simulink model "Signal_Generator"  (R2018a)
settings: Solver=VariableStepAuto  StartTime=0.0  StopTime=0.5  RelTol=1e-3
libraries: simulink x20, commrflib2 x4, commsynccomp2 x3
settings Model: Creator=Alam  LastModifiedBy=Administrator
settings CodeAppCC: StateflowObjectComments=on
settings SimscapeCC: SimscapeNormalizeSystem=off

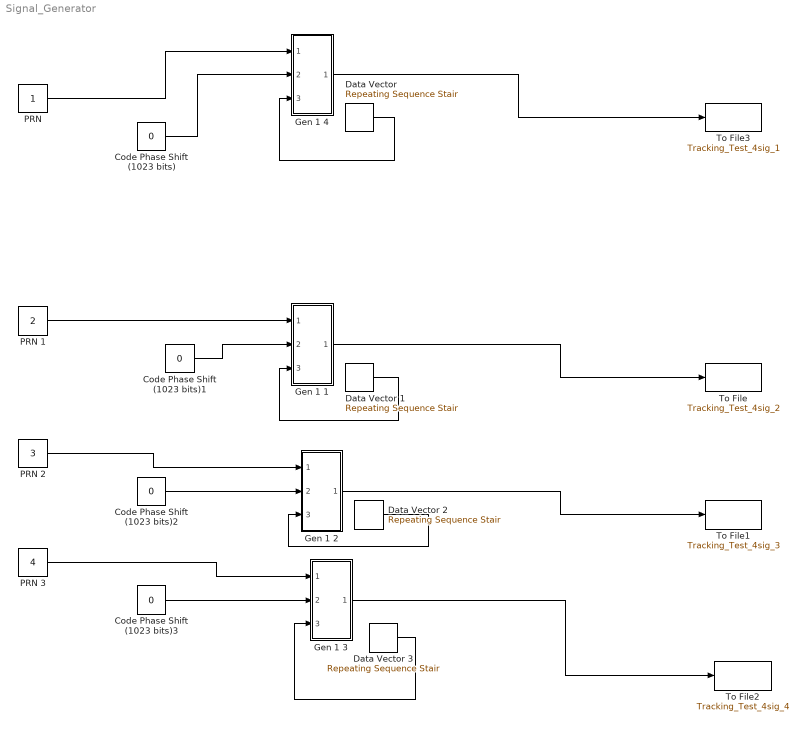
== system Signal_Generator ==
  Code Phase Shift (1023 bits){,1..3} (4 alike) : Constant  Value=0
  Data Vector : simulink/Sources/Repeating Sequence Stair  OutValues=[1 0 0 1 1].'  tsamp=0.1  OutMin=[]  OutMax=[]  OutDataTypeStr=double  OutputDataTypeScalingMode=double  OutDataType=fixdt(0,8)  ConRadixGroup=Best Precision: Vector-wise  OutScaling=2^-12
  Data Vector 1 : simulink/Sources/Repeating Sequence Stair  OutValues=[1 0 1 0 1].'  tsamp=0.1  OutMin=[]  OutMax=[]  OutDataTypeStr=double  OutputDataTypeScalingMode=double  OutDataType=fixdt(0,8)  ConRadixGroup=Best Precision: Vector-wise  OutScaling=2^-12
  Data Vector 2 : simulink/Sources/Repeating Sequence Stair  OutValues=[0 1 1 0 0].'  tsamp=0.1  OutMin=[]  OutMax=[]  OutDataTypeStr=double  OutputDataTypeScalingMode=double  OutDataType=fixdt(0,8)  ConRadixGroup=Best Precision: Vector-wise  OutScaling=2^-12
  Data Vector 3 : simulink/Sources/Repeating Sequence Stair  OutValues=[1 0 0 1 0].'  tsamp=0.1  OutMin=[]  OutMax=[]  OutDataTypeStr=double  OutputDataTypeScalingMode=double  OutDataType=fixdt(0,8)  ConRadixGroup=Best Precision: Vector-wise  OutScaling=2^-12
  Gen 1 1 : Subsystem
  Gen 1 2 : Subsystem
  Gen 1 3 : Subsystem
  Gen 1 4 : Subsystem
  "PRN " : Constant
  PRN 1 : Constant  Value=2
  PRN 2 : Constant  Value=3
  PRN 3 : Constant  Value=4
  To File : ToFile  Filename=Tracking_Test_4sig_2  MatrixName=Tracking_Test_4sig_2  SaveFormat=Timeseries
  To File1 : ToFile  Filename=Tracking_Test_4sig_3  MatrixName=Tracking_Test_4sig_3  SaveFormat=Timeseries
  To File2 : ToFile  Filename=Tracking_Test_4sig_4  MatrixName=Tracking_Test_4sig_4  SaveFormat=Timeseries
  To File3 : ToFile  Filename=Tracking_Test_4sig_1  MatrixName=Tracking_Test_4sig_1  SaveFormat=Timeseries
  wires:
  Gen 1 3/1(Out1) -> To File2/1
  "PRN "/1 -> Gen 1 4/1(In1)
  Gen 1 2/1(Out1) -> To File1/1
  Gen 1 4/1(Out1) -> To File3/1
  Code Phase Shift (1023 bits)/1 -> Gen 1 4/2(In3)
  PRN 1/1 -> Gen 1 1/1(In1)
  Code Phase Shift (1023 bits)1/1 -> Gen 1 1/2(In3)
  PRN 2/1 -> Gen 1 2/1(In1)
  Code Phase Shift (1023 bits)2/1 -> Gen 1 2/2(In3)
  PRN 3/1 -> Gen 1 3/1(In1)
  Code Phase Shift (1023 bits)3/1 -> Gen 1 3/2(In3)
  Data Vector/1 -> Gen 1 4/3("Data ")
  Data Vector 1/1 -> Gen 1 1/3("Data ")
  Data Vector 3/1 -> Gen 1 3/3("Data ")
  Data Vector 2/1 -> Gen 1 2/3("Data ")
  Gen 1 1/1(Out1) -> To File/1

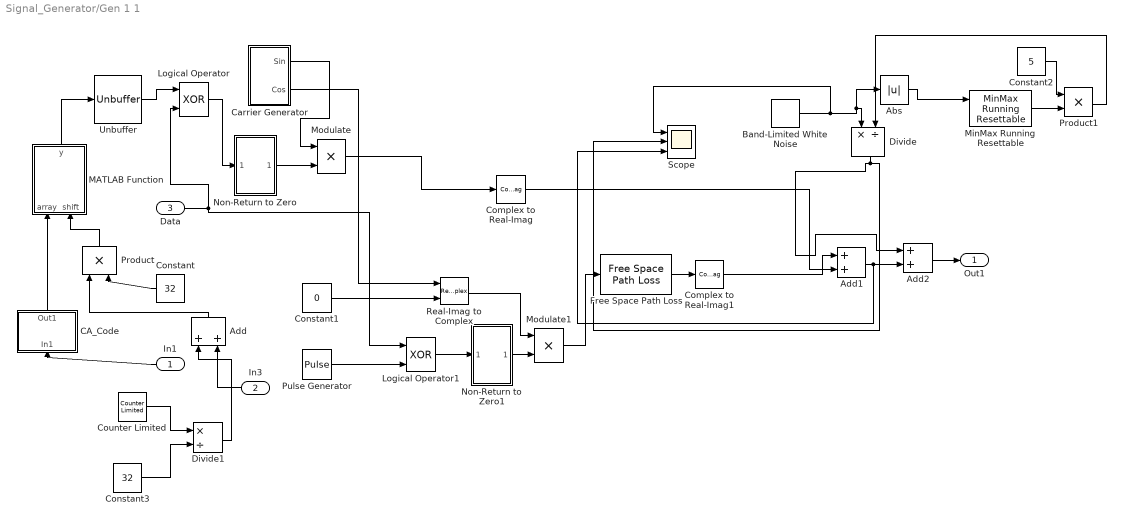
== system Signal_Generator/Gen 1 1 ==
  In1 : Inport
  In3 : Inport  Port=2
  "Data " : Inport  Port=3
  Abs : Abs
  Add : Sum
  Add1 : Sum
  Add2 : Sum
  Band-Limited White Noise : simulink/Sources/Band-Limited White Noise  Cov=[0.4]  Ts=(1/100)*(2*pi/9207000)  seed=[1]
  "CA_Code " : Subsystem
  Carrier Generator : Subsystem
  Complex to Real-Imag : ComplexToRealImag  Output=Real
  Complex to Real-Imag1 : ComplexToRealImag  Output=Real
  Constant : Constant  Value=32
  Constant1 : Constant  Value=0
  Constant2 : Constant  Value=5
  Constant3 : Constant  Value=32
  Counter Limited : simulink/Sources/Counter Limited  uplimit=2^32  tsamp=0.01
  Divide : Product  Inputs=*/
  Divide1 : Product  Inputs=*/
  Free Space Path Loss : commrflib2/Free Space Path Loss  mode=Decibels  dB=3  d=0.100  fc=1920
      settings: SourceProductName=Communications System Toolbox  SourceProductBaseCode=CM
  Logical Operator : Logic  Operator=XOR  AllPortsSameDT=off  OutDataTypeStr=boolean
  Logical Operator1 : Logic  Operator=XOR  AllPortsSameDT=off  OutDataTypeStr=boolean
  MATLAB Function : MATLAB Function  TreatAsAtomicUnit=on
  MinMax Running Resettable : simulink/Math Operations/MinMax Running Resettable  Function=max  vinit=10000
  Modulate : Product
  Modulate1 : Product
  Non-Return to Zero : Subsystem
  Non-Return to Zero1 : Subsystem
  Product : Product
  Product1 : Product
  Pulse Generator : DiscretePulseGenerator  PulseType=Time based  Period=2/10230000  PulseWidth=50
  Real-Imag to Complex : RealImagToComplex
  Scope : Scope  NumInputPorts=3
  Unbuffer : Unbuffer
  Out1 : Outport
  wires:
  In1/1 -> "CA_Code "/1(In1)
  Logical Operator/1 -> Non-Return to Zero/1(In1)
  Non-Return to Zero/1(Out1) -> Modulate/2
  Unbuffer/1 -> Logical Operator/1
  Modulate/1 -> Complex to Real-Imag/1
  "CA_Code "/1(Out1) -> MATLAB Function/1(array)
  MATLAB Function/1(y) -> Unbuffer/1
  Product/1 -> MATLAB Function/2(shift)
  Constant/1 -> Product/2
  Carrier Generator/1(Sin) -> Modulate/1
  "Data "/1 -> Logical Operator1/1, Logical Operator/2
  Pulse Generator/1 -> Logical Operator1/2
  Logical Operator1/1 -> Non-Return to Zero1/1(In1)
  Non-Return to Zero1/1(Out1) -> Modulate1/2
  Modulate1/1 -> Free Space Path Loss/1
  Complex to Real-Imag/1 -> Add1/2
  Free Space Path Loss/1 -> Complex to Real-Imag1/1
  Real-Imag to Complex/1 -> Modulate1/1
  Constant1/1 -> Real-Imag to Complex/2
  Band-Limited White Noise/1 -> Scope/1, Abs/1, Divide/1
  Abs/1 -> MinMax Running Resettable/1
  Divide/1 -> Add2/1, Scope/2
  MinMax Running Resettable/1 -> Product1/2
  Constant2/1 -> Product1/1
  Product1/1 -> Divide/2
  Complex to Real-Imag1/1 -> Add1/1
  Add1/1 -> Scope/3, Add2/2
  Add2/1 -> Out1/1
  Add/1 -> Product/1
  In3/1 -> Add/2
  Counter Limited/1 -> Divide1/1
  Constant3/1 -> Divide1/2
  Divide1/1 -> Add/1
  Carrier Generator/2(Cos) -> Real-Imag to Complex/1

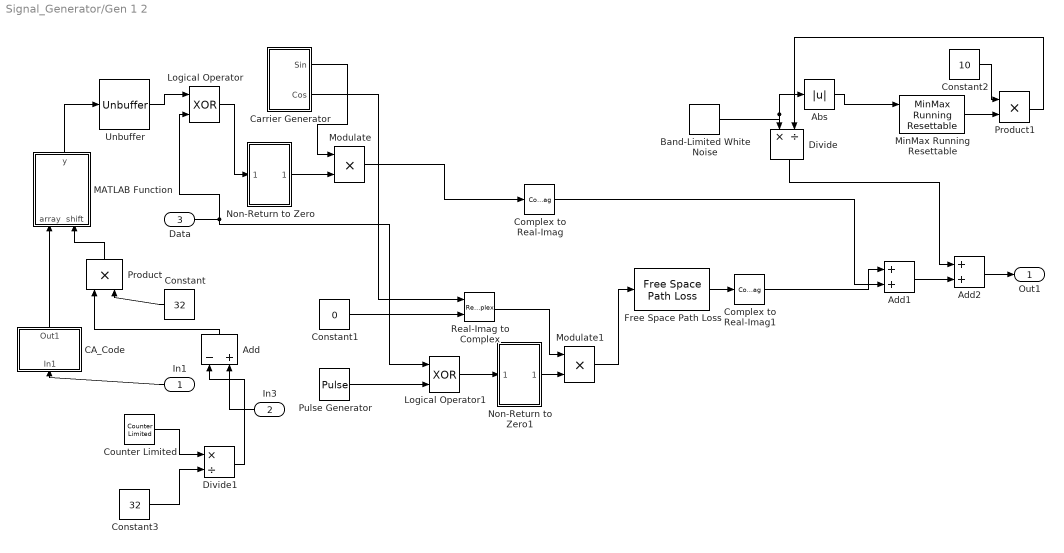
== system Signal_Generator/Gen 1 2 ==
  In1 : Inport
  In3 : Inport  Port=2
  "Data " : Inport  Port=3
  Abs : Abs
  Add : Sum  Inputs=-+
  Add1 : Sum
  Add2 : Sum
  Band-Limited White Noise : simulink/Sources/Band-Limited White Noise  Cov=[0.1]  Ts=(1/100)*(2*pi/9207000)  seed=[1]
  "CA_Code " : Subsystem
  "Carrier Generator " : Subsystem
  Complex to Real-Imag : ComplexToRealImag  Output=Real
  Complex to Real-Imag1 : ComplexToRealImag  Output=Real
  Constant : Constant  Value=32
  Constant1 : Constant  Value=0
  Constant2 : Constant  Value=10
  Constant3 : Constant  Value=32
  Counter Limited : simulink/Sources/Counter Limited  uplimit=2^32  tsamp=0.01
  Divide : Product  Inputs=*/
  Divide1 : Product  Inputs=*/
  Free Space Path Loss : commrflib2/Free Space Path Loss  mode=Decibels  dB=3  d=0.100  fc=1920
      settings: SourceProductName=Communications System Toolbox  SourceProductBaseCode=CM
  Logical Operator : Logic  Operator=XOR  AllPortsSameDT=off  OutDataTypeStr=boolean
  Logical Operator1 : Logic  Operator=XOR  AllPortsSameDT=off  OutDataTypeStr=boolean
  MATLAB Function : MATLAB Function  TreatAsAtomicUnit=on
  MinMax Running Resettable : simulink/Math Operations/MinMax Running Resettable  Function=max  vinit=10000
  Modulate : Product
  Modulate1 : Product
  Non-Return to Zero : Subsystem
  Non-Return to Zero1 : Subsystem
  Product : Product
  Product1 : Product
  Pulse Generator : DiscretePulseGenerator  PulseType=Time based  Period=2/10230000  PulseWidth=50
  Real-Imag to Complex : RealImagToComplex
  Unbuffer : Unbuffer
  Out1 : Outport
  wires:
  In1/1 -> "CA_Code "/1(In1)
  Logical Operator/1 -> Non-Return to Zero/1(In1)
  Non-Return to Zero/1(Out1) -> Modulate/2
  Unbuffer/1 -> Logical Operator/1
  Modulate/1 -> Complex to Real-Imag/1
  "CA_Code "/1(Out1) -> MATLAB Function/1(array)
  MATLAB Function/1(y) -> Unbuffer/1
  Product/1 -> MATLAB Function/2(shift)
  Constant/1 -> Product/2
  "Carrier Generator "/1(Sin) -> Modulate/1
  "Data "/1 -> Logical Operator1/1, Logical Operator/2
  Pulse Generator/1 -> Logical Operator1/2
  Logical Operator1/1 -> Non-Return to Zero1/1(In1)
  Non-Return to Zero1/1(Out1) -> Modulate1/2
  Modulate1/1 -> Free Space Path Loss/1
  Complex to Real-Imag/1 -> Add1/2
  Free Space Path Loss/1 -> Complex to Real-Imag1/1
  Real-Imag to Complex/1 -> Modulate1/1
  Constant1/1 -> Real-Imag to Complex/2
  Complex to Real-Imag1/1 -> Add1/1
  Add1/1 -> Add2/2
  Add2/1 -> Out1/1
  Add/1 -> Product/1
  In3/1 -> Add/2
  Counter Limited/1 -> Divide1/1
  Constant3/1 -> Divide1/2
  Divide1/1 -> Add/1
  "Carrier Generator "/2(Cos) -> Real-Imag to Complex/1
  Abs/1 -> MinMax Running Resettable/1
  Constant2/1 -> Product1/1
  Band-Limited White Noise/1 -> Abs/1, Divide/1
  Product1/1 -> Divide/2
  MinMax Running Resettable/1 -> Product1/2
  Divide/1 -> Add2/1

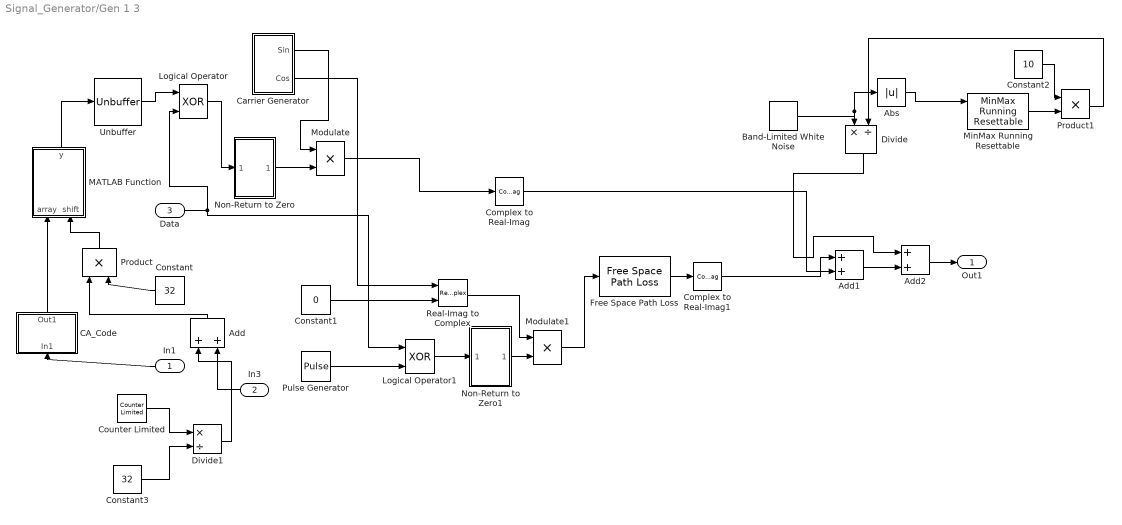
== system Signal_Generator/Gen 1 3 ==
  In1 : Inport
  In3 : Inport  Port=2
  "Data " : Inport  Port=3
  Abs : Abs
  Add : Sum
  Add1 : Sum
  Add2 : Sum
  Band-Limited White Noise : simulink/Sources/Band-Limited White Noise  Cov=[0.1]  Ts=(1/100)*(2*pi/9207000)  seed=[1]
  "CA_Code " : Subsystem
  "Carrier Generator " : Subsystem
  Complex to Real-Imag : ComplexToRealImag  Output=Real
  Complex to Real-Imag1 : ComplexToRealImag  Output=Real
  Constant : Constant  Value=32
  Constant1 : Constant  Value=0
  Constant2 : Constant  Value=10
  Constant3 : Constant  Value=32
  Counter Limited : simulink/Sources/Counter Limited  uplimit=2^32  tsamp=0.01
  Divide : Product  Inputs=*/
  Divide1 : Product  Inputs=*/
  Free Space Path Loss : commrflib2/Free Space Path Loss  mode=Decibels  dB=3  d=0.100  fc=1920
      settings: SourceProductName=Communications System Toolbox  SourceProductBaseCode=CM
  Logical Operator : Logic  Operator=XOR  AllPortsSameDT=off  OutDataTypeStr=boolean
  Logical Operator1 : Logic  Operator=XOR  AllPortsSameDT=off  OutDataTypeStr=boolean
  MATLAB Function : MATLAB Function  TreatAsAtomicUnit=on
  MinMax Running Resettable : simulink/Math Operations/MinMax Running Resettable  Function=max  vinit=10000
  Modulate : Product
  Modulate1 : Product
  Non-Return to Zero : Subsystem
  Non-Return to Zero1 : Subsystem
  Product : Product
  Product1 : Product
  Pulse Generator : DiscretePulseGenerator  PulseType=Time based  Period=2/10230000  PulseWidth=50
  Real-Imag to Complex : RealImagToComplex
  Unbuffer : Unbuffer
  Out1 : Outport
  wires:
  In1/1 -> "CA_Code "/1(In1)
  Logical Operator/1 -> Non-Return to Zero/1(In1)
  Non-Return to Zero/1(Out1) -> Modulate/2
  Unbuffer/1 -> Logical Operator/1
  Modulate/1 -> Complex to Real-Imag/1
  "CA_Code "/1(Out1) -> MATLAB Function/1(array)
  MATLAB Function/1(y) -> Unbuffer/1
  Product/1 -> MATLAB Function/2(shift)
  Constant/1 -> Product/2
  "Carrier Generator "/1(Sin) -> Modulate/1
  "Data "/1 -> Logical Operator1/1, Logical Operator/2
  Pulse Generator/1 -> Logical Operator1/2
  Logical Operator1/1 -> Non-Return to Zero1/1(In1)
  Non-Return to Zero1/1(Out1) -> Modulate1/2
  Modulate1/1 -> Free Space Path Loss/1
  Complex to Real-Imag/1 -> Add1/2
  Free Space Path Loss/1 -> Complex to Real-Imag1/1
  Real-Imag to Complex/1 -> Modulate1/1
  Constant1/1 -> Real-Imag to Complex/2
  Band-Limited White Noise/1 -> Abs/1, Divide/1
  Abs/1 -> MinMax Running Resettable/1
  Divide/1 -> Add2/1
  MinMax Running Resettable/1 -> Product1/2
  Constant2/1 -> Product1/1
  Product1/1 -> Divide/2
  Complex to Real-Imag1/1 -> Add1/1
  Add1/1 -> Add2/2
  Add2/1 -> Out1/1
  Add/1 -> Product/1
  In3/1 -> Add/2
  Counter Limited/1 -> Divide1/1
  Constant3/1 -> Divide1/2
  Divide1/1 -> Add/1
  "Carrier Generator "/2(Cos) -> Real-Imag to Complex/1

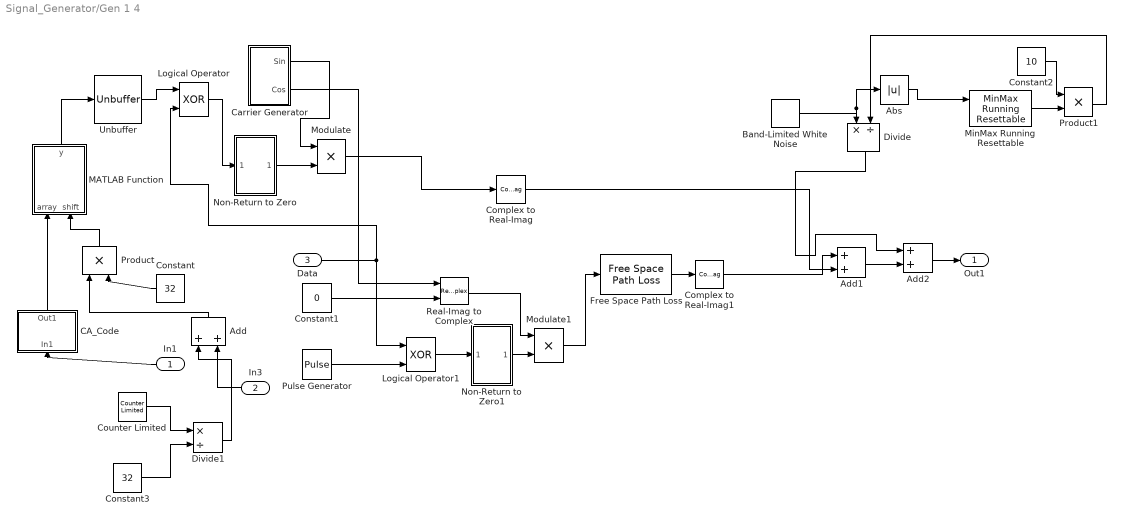
== system Signal_Generator/Gen 1 4 ==
  In1 : Inport
  In3 : Inport  Port=2
  "Data " : Inport  Port=3
  Abs : Abs
  Add : Sum
  Add1 : Sum
  Add2 : Sum
  Band-Limited White Noise : simulink/Sources/Band-Limited White Noise  Cov=[0.1]  Ts=(1/100)*(2*pi/9207000)  seed=[1]
  "CA_Code " : Subsystem
  "Carrier Generator " : Subsystem
  Complex to Real-Imag : ComplexToRealImag  Output=Real
  Complex to Real-Imag1 : ComplexToRealImag  Output=Real
  Constant : Constant  Value=32
  Constant1 : Constant  Value=0
  Constant2 : Constant  Value=10
  Constant3 : Constant  Value=32
  Counter Limited : simulink/Sources/Counter Limited  uplimit=2^32  tsamp=0.01
  Divide : Product  Inputs=*/
  Divide1 : Product  Inputs=*/
  Free Space Path Loss : commrflib2/Free Space Path Loss  mode=Decibels  dB=3  d=0.100  fc=1920
      settings: SourceProductName=Communications System Toolbox  SourceProductBaseCode=CM
  Logical Operator : Logic  Operator=XOR  AllPortsSameDT=off  OutDataTypeStr=boolean
  Logical Operator1 : Logic  Operator=XOR  AllPortsSameDT=off  OutDataTypeStr=boolean
  MATLAB Function : MATLAB Function  TreatAsAtomicUnit=on
  MinMax Running Resettable : simulink/Math Operations/MinMax Running Resettable  Function=max  vinit=10000
  Modulate : Product
  Modulate1 : Product
  Non-Return to Zero : Subsystem
  Non-Return to Zero1 : Subsystem
  Product : Product
  Product1 : Product
  Pulse Generator : DiscretePulseGenerator  PulseType=Time based  Period=2/10230000  PulseWidth=50
  Real-Imag to Complex : RealImagToComplex
  Unbuffer : Unbuffer
  Out1 : Outport
  wires:
  In1/1 -> "CA_Code "/1(In1)
  Logical Operator/1 -> Non-Return to Zero/1(In1)
  Non-Return to Zero/1(Out1) -> Modulate/2
  Unbuffer/1 -> Logical Operator/1
  Modulate/1 -> Complex to Real-Imag/1
  "CA_Code "/1(Out1) -> MATLAB Function/1(array)
  MATLAB Function/1(y) -> Unbuffer/1
  Product/1 -> MATLAB Function/2(shift)
  Constant/1 -> Product/2
  "Carrier Generator "/1(Sin) -> Modulate/1
  "Data "/1 -> Logical Operator/2, Logical Operator1/1
  Pulse Generator/1 -> Logical Operator1/2
  Logical Operator1/1 -> Non-Return to Zero1/1(In1)
  Non-Return to Zero1/1(Out1) -> Modulate1/2
  Modulate1/1 -> Free Space Path Loss/1
  Complex to Real-Imag/1 -> Add1/2
  Free Space Path Loss/1 -> Complex to Real-Imag1/1
  Real-Imag to Complex/1 -> Modulate1/1
  Constant1/1 -> Real-Imag to Complex/2
  Band-Limited White Noise/1 -> Abs/1, Divide/1
  Abs/1 -> MinMax Running Resettable/1
  Divide/1 -> Add2/1
  MinMax Running Resettable/1 -> Product1/2
  Constant2/1 -> Product1/1
  Product1/1 -> Divide/2
  Complex to Real-Imag1/1 -> Add1/1
  Add1/1 -> Add2/2
  Add2/1 -> Out1/1
  Add/1 -> Product/1
  In3/1 -> Add/2
  Counter Limited/1 -> Divide1/1
  Constant3/1 -> Divide1/2
  Divide1/1 -> Add/1
  "Carrier Generator "/2(Cos) -> Real-Imag to Complex/1

== system Signal_Generator/Gen 1 1/CA_Code  ==
  In1 : Inport
  CA_Code : MATLAB Function  TreatAsAtomicUnit=on  SystemSampleTime=0.001
  Constant1 : Constant  Value=32
  Reshape : Reshape  OutputDimensionality=Column vector (2-D)
  Out1 : Outport
  wires:
  In1/1 -> CA_Code/1(sv)
  CA_Code/1(g) -> Reshape/1
  Constant1/1 -> CA_Code/2(fs)
  Reshape/1 -> Out1/1

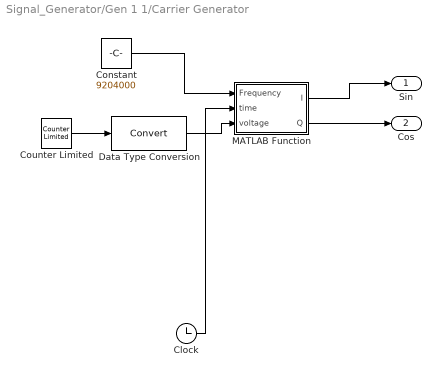
== system Signal_Generator/Gen 1 1/Carrier Generator ==
  Clock : Clock
  Constant : Constant  Value=9204000
  Counter Limited : simulink/Sources/Counter Limited  uplimit=2500  tsamp=1/2500
  Data Type Conversion : DataTypeConversion
  MATLAB Function : MATLAB Function  TreatAsAtomicUnit=on
  Sin : Outport
  Cos : Outport  Port=2
  wires:
  MATLAB Function/1(I) -> Sin/1
  Counter Limited/1 -> Data Type Conversion/1
  Data Type Conversion/1 -> MATLAB Function/3(voltage)
  Clock/1 -> MATLAB Function/2(time)
  Constant/1 -> MATLAB Function/1(Frequency)
  MATLAB Function/2(Q) -> Cos/1

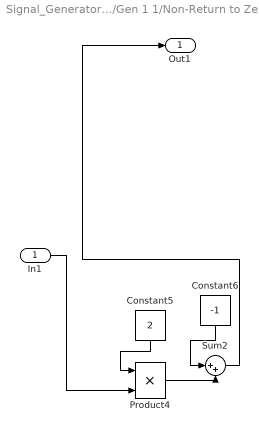
== system Signal_Generator/Gen 1 1/Non-Return to Zero ==
  In1 : Inport
  Constant5 : Constant  Value=2  SampleTime=1.52587891e-8
  Constant6 : Constant  Value=-1
  Product4 : Product
  Sum2 : Sum  Inputs=|++
  Out1 : Outport
  wires:
  Product4/1 -> Sum2/2
  Constant5/1 -> Product4/1
  Sum2/1 -> Out1/1
  Constant6/1 -> Sum2/1
  In1/1 -> Product4/2

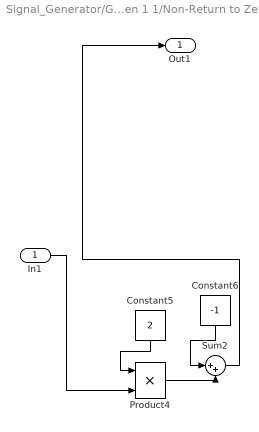
== system Signal_Generator/Gen 1 1/Non-Return to Zero1 ==
  In1 : Inport
  Constant5 : Constant  Value=2  SampleTime=1.52587891e-8
  Constant6 : Constant  Value=-1
  Product4 : Product
  Sum2 : Sum  Inputs=|++
  Out1 : Outport
  wires:
  Product4/1 -> Sum2/2
  Constant5/1 -> Product4/1
  Sum2/1 -> Out1/1
  Constant6/1 -> Sum2/1
  In1/1 -> Product4/2

== system Signal_Generator/Gen 1 2/CA_Code  ==
  In1 : Inport
  CA_Code : MATLAB Function  TreatAsAtomicUnit=on  SystemSampleTime=0.001
  Constant1 : Constant  Value=32
  Reshape : Reshape  OutputDimensionality=Column vector (2-D)
  Out1 : Outport
  wires:
  In1/1 -> CA_Code/1(sv)
  CA_Code/1(g) -> Reshape/1
  Constant1/1 -> CA_Code/2(fs)
  Reshape/1 -> Out1/1

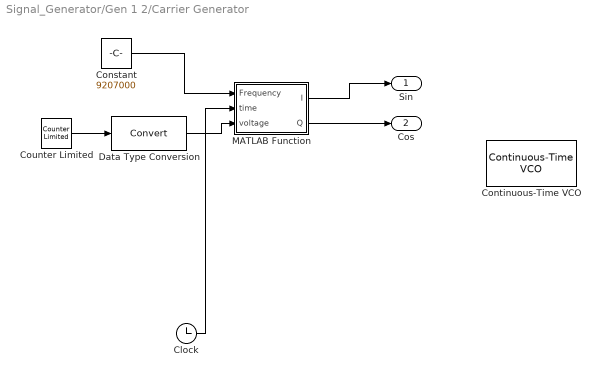
== system Signal_Generator/Gen 1 2/Carrier Generator  ==
  Clock : Clock
  Constant : Constant  Value=9207000
  Continuous-Time VCO : commsynccomp2/Continuous-Time VCO  Ac=1  Fc=9207000  Kc=0.04  Ph=0
      settings: SourceProductName=Communications System Toolbox  SourceProductBaseCode=CM
  Counter Limited : simulink/Sources/Counter Limited  uplimit=2500  tsamp=1/2500
  Data Type Conversion : DataTypeConversion
  MATLAB Function : MATLAB Function  TreatAsAtomicUnit=on
  Sin : Outport
  Cos : Outport  Port=2
  wires:
  MATLAB Function/1(I) -> Sin/1
  Counter Limited/1 -> Data Type Conversion/1
  Data Type Conversion/1 -> MATLAB Function/3(voltage)
  Clock/1 -> MATLAB Function/2(time)
  Constant/1 -> MATLAB Function/1(Frequency)
  MATLAB Function/2(Q) -> Cos/1

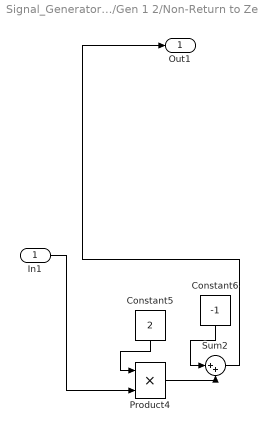
== system Signal_Generator/Gen 1 2/Non-Return to Zero ==
  In1 : Inport
  Constant5 : Constant  Value=2  SampleTime=1.52587891e-8
  Constant6 : Constant  Value=-1
  Product4 : Product
  Sum2 : Sum  Inputs=|++
  Out1 : Outport
  wires:
  Product4/1 -> Sum2/2
  Constant5/1 -> Product4/1
  Sum2/1 -> Out1/1
  Constant6/1 -> Sum2/1
  In1/1 -> Product4/2

== system Signal_Generator/Gen 1 2/Non-Return to Zero1 ==
  In1 : Inport
  Constant5 : Constant  Value=2  SampleTime=1.52587891e-8
  Constant6 : Constant  Value=-1
  Product4 : Product
  Sum2 : Sum  Inputs=|++
  Out1 : Outport
  wires:
  Product4/1 -> Sum2/2
  Constant5/1 -> Product4/1
  Sum2/1 -> Out1/1
  Constant6/1 -> Sum2/1
  In1/1 -> Product4/2

== system Signal_Generator/Gen 1 3/CA_Code  ==
  In1 : Inport
  CA_Code : MATLAB Function  TreatAsAtomicUnit=on  SystemSampleTime=0.001
  Constant1 : Constant  Value=32
  Reshape : Reshape  OutputDimensionality=Column vector (2-D)
  Out1 : Outport
  wires:
  In1/1 -> CA_Code/1(sv)
  CA_Code/1(g) -> Reshape/1
  Constant1/1 -> CA_Code/2(fs)
  Reshape/1 -> Out1/1

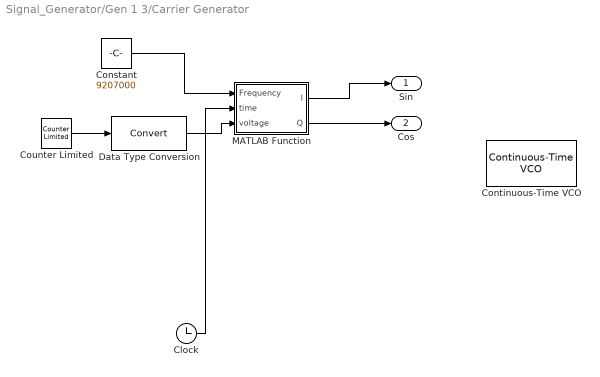
== system Signal_Generator/Gen 1 3/Carrier Generator  ==
  Clock : Clock
  Constant : Constant  Value=9207000
  Continuous-Time VCO : commsynccomp2/Continuous-Time VCO  Ac=1  Fc=9207000  Kc=0.04  Ph=0
      settings: SourceProductName=Communications System Toolbox  SourceProductBaseCode=CM
  Counter Limited : simulink/Sources/Counter Limited  uplimit=2500  tsamp=1/2500
  Data Type Conversion : DataTypeConversion
  MATLAB Function : MATLAB Function  TreatAsAtomicUnit=on
  Sin : Outport
  Cos : Outport  Port=2
  wires:
  MATLAB Function/1(I) -> Sin/1
  Counter Limited/1 -> Data Type Conversion/1
  Data Type Conversion/1 -> MATLAB Function/3(voltage)
  Clock/1 -> MATLAB Function/2(time)
  Constant/1 -> MATLAB Function/1(Frequency)
  MATLAB Function/2(Q) -> Cos/1

== system Signal_Generator/Gen 1 3/Non-Return to Zero ==
  In1 : Inport
  Constant5 : Constant  Value=2  SampleTime=1.52587891e-8
  Constant6 : Constant  Value=-1
  Product4 : Product
  Sum2 : Sum  Inputs=|++
  Out1 : Outport
  wires:
  Product4/1 -> Sum2/2
  Constant5/1 -> Product4/1
  Sum2/1 -> Out1/1
  Constant6/1 -> Sum2/1
  In1/1 -> Product4/2

== system Signal_Generator/Gen 1 3/Non-Return to Zero1 ==
  In1 : Inport
  Constant5 : Constant  Value=2  SampleTime=1.52587891e-8
  Constant6 : Constant  Value=-1
  Product4 : Product
  Sum2 : Sum  Inputs=|++
  Out1 : Outport
  wires:
  Product4/1 -> Sum2/2
  Constant5/1 -> Product4/1
  Sum2/1 -> Out1/1
  Constant6/1 -> Sum2/1
  In1/1 -> Product4/2

== system Signal_Generator/Gen 1 4/CA_Code  ==
  In1 : Inport
  CA_Code : MATLAB Function  TreatAsAtomicUnit=on  SystemSampleTime=0.001
  Constant1 : Constant  Value=32
  Reshape : Reshape  OutputDimensionality=Column vector (2-D)
  Out1 : Outport
  wires:
  In1/1 -> CA_Code/1(sv)
  CA_Code/1(g) -> Reshape/1
  Constant1/1 -> CA_Code/2(fs)
  Reshape/1 -> Out1/1

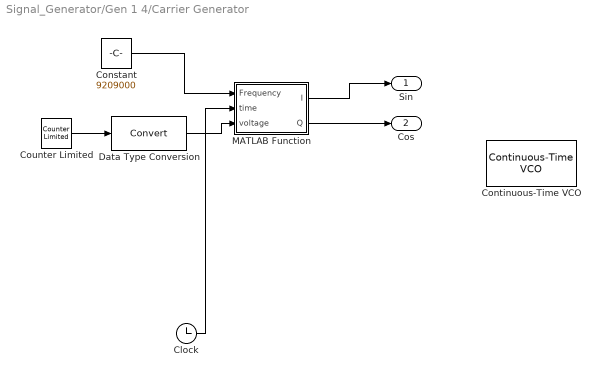
== system Signal_Generator/Gen 1 4/Carrier Generator  ==
  Clock : Clock
  Constant : Constant  Value=9209000
  Continuous-Time VCO : commsynccomp2/Continuous-Time VCO  Ac=1  Fc=9207000  Kc=0.04  Ph=0
      settings: SourceProductName=Communications System Toolbox  SourceProductBaseCode=CM
  Counter Limited : simulink/Sources/Counter Limited  uplimit=2500  tsamp=1/2500
  Data Type Conversion : DataTypeConversion
  MATLAB Function : MATLAB Function  TreatAsAtomicUnit=on
  Sin : Outport
  Cos : Outport  Port=2
  wires:
  MATLAB Function/1(I) -> Sin/1
  Counter Limited/1 -> Data Type Conversion/1
  Data Type Conversion/1 -> MATLAB Function/3(voltage)
  Clock/1 -> MATLAB Function/2(time)
  Constant/1 -> MATLAB Function/1(Frequency)
  MATLAB Function/2(Q) -> Cos/1

== system Signal_Generator/Gen 1 4/Non-Return to Zero ==
  In1 : Inport
  Constant5 : Constant  Value=2  SampleTime=1.52587891e-8
  Constant6 : Constant  Value=-1
  Product4 : Product
  Sum2 : Sum  Inputs=|++
  Out1 : Outport
  wires:
  Product4/1 -> Sum2/2
  Constant5/1 -> Product4/1
  Sum2/1 -> Out1/1
  Constant6/1 -> Sum2/1
  In1/1 -> Product4/2

== system Signal_Generator/Gen 1 4/Non-Return to Zero1 ==
  In1 : Inport
  Constant5 : Constant  Value=2  SampleTime=1.52587891e-8
  Constant6 : Constant  Value=-1
  Product4 : Product
  Sum2 : Sum  Inputs=|++
  Out1 : Outport
  wires:
  Product4/1 -> Sum2/2
  Constant5/1 -> Product4/1
  Sum2/1 -> Out1/1
  Constant6/1 -> Sum2/1
  In1/1 -> Product4/2

== matlab function Signal_Generator/Gen 1 2/CA_Code /CA_Code ==
  data: sv input; g output; fs input
function g=CAcode(sv,fs)
coder.extrinsic('warning')
% function G=CACODE(SV,FS) 
% Generates 1023 length C/A Codes for GPS PRNs 1-37
%
% 
% g: nx1023 matrix- with each PRN in each row with symbols 1 and 0
% sv: a row or column vector of the SV's to be generated
% 	 valid entries are 1 to 37
% fs: optional number of samples per chip (defaults to 1), fractional samples allowed, must be 1 or greater.
%
% For multiple samples per chip, function is a zero order hold. 
%
%
% For example to generate the C/A codes for PRN 6 and PRN 12 use:
% g=cacode([6 12]),
% and to generate the C/A codes for PRN 6 and PRN 12 at 5 MHz use
% g=cacode([6 12],5/1.023)
% 
%
% For more information refer to the "GPS SPS Signal Specification"
% http://www.navcen.uscg.gov/pubs/gps/sigspec/default.htm
%
% Dan Boschen 12-30-2007
% boschen@loglin.com

% Revision History
% rev 1.0 Dan Boschen 4-15-2007  Initial Release
%
% rev 1.1 Dan Boschen 7-15-2007  Corrected error with taps for PRN30, should be [2,7] was 
% 					incorrect as [1 7]. Thank you Jadah Zak for finding this.
%
%
% rev 1.2 Dan Boschen 12-26-2007 Fixed column index error when ceil ~ L 
%				Thank you Jared Meadows for finding this.
%
% rev 1.3 Dan Boschen 12-30-2007 Changed comment "first order hold" to
% "zero order hold".
%
% rev 1.4 Dan Boschen 6-1-2010   Updated email address in comments



if nargin<2
	fs=1;
end


if (max(sv)>37) || (min(sv)<1) || (min(size(sv))~=1)
	error('sv must be a row or column vector with integers between 1 and 37\n')
end

if fs<1
	error('fs must be 1 or greater\n')
end	

% force integers
testint=round(sv)-sv;
if testint ~= 0 
	warning('non-integer value entered for sv, rounding to closest integer\n');
	sv = round(sv);
end


% table of C/A Code Tap Selection (sets delay for G2 generator)
tap=[2 6;
    3 7;
    4 8;
    5 9;
    1 9;
    2 10;
    1 8;
    2 9;
    3 10;
    2 3;
    3 4;
    5 6;
    6 7;
    7 8;
    8 9;
    9 10;
    1 4;
    2 5;
    3 6;
    4 7;
    5 8;
    6 9;
    1 3;
    4 6;
    5 7;
    6 8;
    7 9;
    8 10;
    1 6;
    2 7;
    3 8;
    4 9
    5 10
    4 10
    1 7
    2 8
    4 10];

% G1 LFSR: x^10+x^3+1
s=[0 0 1 0 0 0 0 0 0 1];
n=length(s);
g1=ones(1,n);	%initialization vector for G1

%g=ones(1,38192);
%g2=ones(1,38192);
%gfs=ones(1,38192);

g=ones(1,65536/2);
g2=ones(1,65536/2);
gfs=ones(1,65536/2);

L=2^n-1;

% G2j LFSR: x^10+x^9+x^8+x^6+x^3+x^2+1
t=[0 1 1 0 0 1 0 1 1 1];
q=ones(1,n);	%initialization vector for G2

% generate C/A Code sequences:
tap_sel=tap(sv,:);
for inc=1:L
    g2(:,inc)=mod(sum(q(tap_sel),2),2);
    g(:,inc)=mod(g1(n)+g2(:,inc),2);
   g1=[mod(sum(g1.*s),2) g1(1:n-1)];
   q=[mod(sum(q.*t),2) q(1:n-1)];
end

%upsample to desired rate
if fs~=1
	%fractional upsampling with zero order hold
	index=0;
	for cnt = 1/fs:1/fs:L
		index=index+1;
		if ceil(cnt) > L   %traps a floating point error in index
			gfs(:,index)=g(:,L);
		else
			gfs(:,index)=g(:,ceil(cnt));
		end
	end 
	g=gfs;
end

== matlab function Signal_Generator/Gen 1 4/CA_Code /CA_Code ==
  data: sv input; g output; fs input
function g=CAcode(sv,fs)
coder.extrinsic('warning')
% function G=CACODE(SV,FS) 
% Generates 1023 length C/A Codes for GPS PRNs 1-37
%
% 
% g: nx1023 matrix- with each PRN in each row with symbols 1 and 0
% sv: a row or column vector of the SV's to be generated
% 	 valid entries are 1 to 37
% fs: optional number of samples per chip (defaults to 1), fractional samples allowed, must be 1 or greater.
%
% For multiple samples per chip, function is a zero order hold. 
%
%
% For example to generate the C/A codes for PRN 6 and PRN 12 use:
% g=cacode([6 12]),
% and to generate the C/A codes for PRN 6 and PRN 12 at 5 MHz use
% g=cacode([6 12],5/1.023)
% 
%
% For more information refer to the "GPS SPS Signal Specification"
% http://www.navcen.uscg.gov/pubs/gps/sigspec/default.htm
%
% Dan Boschen 12-30-2007
% boschen@loglin.com

% Revision History
% rev 1.0 Dan Boschen 4-15-2007  Initial Release
%
% rev 1.1 Dan Boschen 7-15-2007  Corrected error with taps for PRN30, should be [2,7] was 
% 					incorrect as [1 7]. Thank you Jadah Zak for finding this.
%
%
% rev 1.2 Dan Boschen 12-26-2007 Fixed column index error when ceil ~ L 
%				Thank you Jared Meadows for finding this.
%
% rev 1.3 Dan Boschen 12-30-2007 Changed comment "first order hold" to
% "zero order hold".
%
% rev 1.4 Dan Boschen 6-1-2010   Updated email address in comments



if nargin<2
	fs=1;
end


if (max(sv)>37) || (min(sv)<1) || (min(size(sv))~=1)
	error('sv must be a row or column vector with integers between 1 and 37\n')
end

if fs<1
	error('fs must be 1 or greater\n')
end	

% force integers
testint=round(sv)-sv;
if testint ~= 0 
	warning('non-integer value entered for sv, rounding to closest integer\n');
	sv = round(sv);
end


% table of C/A Code Tap Selection (sets delay for G2 generator)
tap=[2 6;
    3 7;
    4 8;
    5 9;
    1 9;
    2 10;
    1 8;
    2 9;
    3 10;
    2 3;
    3 4;
    5 6;
    6 7;
    7 8;
    8 9;
    9 10;
    1 4;
    2 5;
    3 6;
    4 7;
    5 8;
    6 9;
    1 3;
    4 6;
    5 7;
    6 8;
    7 9;
    8 10;
    1 6;
    2 7;
    3 8;
    4 9
    5 10
    4 10
    1 7
    2 8
    4 10];

% G1 LFSR: x^10+x^3+1
s=[0 0 1 0 0 0 0 0 0 1];
n=length(s);
g1=ones(1,n);	%initialization vector for G1

%g=ones(1,38192);
%g2=ones(1,38192);
%gfs=ones(1,38192);

g=ones(1,65536/2);
g2=ones(1,65536/2);
gfs=ones(1,65536/2);

L=2^n-1;

% G2j LFSR: x^10+x^9+x^8+x^6+x^3+x^2+1
t=[0 1 1 0 0 1 0 1 1 1];
q=ones(1,n);	%initialization vector for G2

% generate C/A Code sequences:
tap_sel=tap(sv,:);
for inc=1:L
    g2(:,inc)=mod(sum(q(tap_sel),2),2);
    g(:,inc)=mod(g1(n)+g2(:,inc),2);
   g1=[mod(sum(g1.*s),2) g1(1:n-1)];
   q=[mod(sum(q.*t),2) q(1:n-1)];
end

%upsample to desired rate
if fs~=1
	%fractional upsampling with zero order hold
	index=0;
	for cnt = 1/fs:1/fs:L
		index=index+1;
		if ceil(cnt) > L   %traps a floating point error in index
			gfs(:,index)=g(:,L);
		else
			gfs(:,index)=g(:,ceil(cnt));
		end
	end 
	g=gfs;
end

== matlab function Signal_Generator/Gen 1 1/CA_Code /CA_Code ==
  data: sv input; g output; fs input
function g=CAcode(sv,fs)
coder.extrinsic('warning')
% function G=CACODE(SV,FS) 
% Generates 1023 length C/A Codes for GPS PRNs 1-37
%
% 
% g: nx1023 matrix- with each PRN in each row with symbols 1 and 0
% sv: a row or column vector of the SV's to be generated
% 	 valid entries are 1 to 37
% fs: optional number of samples per chip (defaults to 1), fractional samples allowed, must be 1 or greater.
%
% For multiple samples per chip, function is a zero order hold. 
%
%
% For example to generate the C/A codes for PRN 6 and PRN 12 use:
% g=cacode([6 12]),
% and to generate the C/A codes for PRN 6 and PRN 12 at 5 MHz use
% g=cacode([6 12],5/1.023)
% 
%
% For more information refer to the "GPS SPS Signal Specification"
% http://www.navcen.uscg.gov/pubs/gps/sigspec/default.htm
%
% Dan Boschen 12-30-2007
% boschen@loglin.com

% Revision History
% rev 1.0 Dan Boschen 4-15-2007  Initial Release
%
% rev 1.1 Dan Boschen 7-15-2007  Corrected error with taps for PRN30, should be [2,7] was 
% 					incorrect as [1 7]. Thank you Jadah Zak for finding this.
%
%
% rev 1.2 Dan Boschen 12-26-2007 Fixed column index error when ceil ~ L 
%				Thank you Jared Meadows for finding this.
%
% rev 1.3 Dan Boschen 12-30-2007 Changed comment "first order hold" to
% "zero order hold".
%
% rev 1.4 Dan Boschen 6-1-2010   Updated email address in comments



if nargin<2
	fs=1;
end


if (max(sv)>37) || (min(sv)<1) || (min(size(sv))~=1)
	error('sv must be a row or column vector with integers between 1 and 37\n')
end

if fs<1
	error('fs must be 1 or greater\n')
end	

% force integers
testint=round(sv)-sv;
if testint ~= 0 
	warning('non-integer value entered for sv, rounding to closest integer\n');
	sv = round(sv);
end


% table of C/A Code Tap Selection (sets delay for G2 generator)
tap=[2 6;
    3 7;
    4 8;
    5 9;
    1 9;
    2 10;
    1 8;
    2 9;
    3 10;
    2 3;
    3 4;
    5 6;
    6 7;
    7 8;
    8 9;
    9 10;
    1 4;
    2 5;
    3 6;
    4 7;
    5 8;
    6 9;
    1 3;
    4 6;
    5 7;
    6 8;
    7 9;
    8 10;
    1 6;
    2 7;
    3 8;
    4 9
    5 10
    4 10
    1 7
    2 8
    4 10];

% G1 LFSR: x^10+x^3+1
s=[0 0 1 0 0 0 0 0 0 1];
n=length(s);
g1=ones(1,n);	%initialization vector for G1

%g=ones(1,38192);
%g2=ones(1,38192);
%gfs=ones(1,38192);

g=ones(1,65536/2);
g2=ones(1,65536/2);
gfs=ones(1,65536/2);

L=2^n-1;

% G2j LFSR: x^10+x^9+x^8+x^6+x^3+x^2+1
t=[0 1 1 0 0 1 0 1 1 1];
q=ones(1,n);	%initialization vector for G2

% generate C/A Code sequences:
tap_sel=tap(sv,:);
for inc=1:L
    g2(:,inc)=mod(sum(q(tap_sel),2),2);
    g(:,inc)=mod(g1(n)+g2(:,inc),2);
   g1=[mod(sum(g1.*s),2) g1(1:n-1)];
   q=[mod(sum(q.*t),2) q(1:n-1)];
end

%upsample to desired rate
if fs~=1
	%fractional upsampling with zero order hold
	index=0;
	for cnt = 1/fs:1/fs:L
		index=index+1;
		if ceil(cnt) > L   %traps a floating point error in index
			gfs(:,index)=g(:,L);
		else
			gfs(:,index)=g(:,ceil(cnt));
		end
	end 
	g=gfs;
end

== matlab function Signal_Generator/Gen 1 2/MATLAB Function ==
  data: array input; y output; shift input
function y = fcn(array, shift)

y = circshift(array, shift);

== matlab function Signal_Generator/Gen 1 4/MATLAB Function ==
  data: array input; y output; shift input
function y = fcn(array, shift)

y = circshift(array, shift);

== matlab function Signal_Generator/Gen 1 1/MATLAB Function ==
  data: array input; y output; shift input
function y = fcn(array, shift)

y = circshift(array, shift);

== matlab function Signal_Generator/Gen 1 3/Carrier Generator /MATLAB Function ==
  data: Frequency input; I output; time input; voltage input; Q output
function [I,Q]= fcn(Frequency, time, voltage)
u=2*pi*(Frequency+0.04*voltage)*time;
I=sin(u);
Q=cos(u);

== matlab function Signal_Generator/Gen 1 3/CA_Code /CA_Code ==
  data: sv input; g output; fs input
function g=CAcode(sv,fs)
coder.extrinsic('warning')
% function G=CACODE(SV,FS) 
% Generates 1023 length C/A Codes for GPS PRNs 1-37
%
% 
% g: nx1023 matrix- with each PRN in each row with symbols 1 and 0
% sv: a row or column vector of the SV's to be generated
% 	 valid entries are 1 to 37
% fs: optional number of samples per chip (defaults to 1), fractional samples allowed, must be 1 or greater.
%
% For multiple samples per chip, function is a zero order hold. 
%
%
% For example to generate the C/A codes for PRN 6 and PRN 12 use:
% g=cacode([6 12]),
% and to generate the C/A codes for PRN 6 and PRN 12 at 5 MHz use
% g=cacode([6 12],5/1.023)
% 
%
% For more information refer to the "GPS SPS Signal Specification"
% http://www.navcen.uscg.gov/pubs/gps/sigspec/default.htm
%
% Dan Boschen 12-30-2007
% boschen@loglin.com

% Revision History
% rev 1.0 Dan Boschen 4-15-2007  Initial Release
%
% rev 1.1 Dan Boschen 7-15-2007  Corrected error with taps for PRN30, should be [2,7] was 
% 					incorrect as [1 7]. Thank you Jadah Zak for finding this.
%
%
% rev 1.2 Dan Boschen 12-26-2007 Fixed column index error when ceil ~ L 
%				Thank you Jared Meadows for finding this.
%
% rev 1.3 Dan Boschen 12-30-2007 Changed comment "first order hold" to
% "zero order hold".
%
% rev 1.4 Dan Boschen 6-1-2010   Updated email address in comments



if nargin<2
	fs=1;
end


if (max(sv)>37) || (min(sv)<1) || (min(size(sv))~=1)
	error('sv must be a row or column vector with integers between 1 and 37\n')
end

if fs<1
	error('fs must be 1 or greater\n')
end	

% force integers
testint=round(sv)-sv;
if testint ~= 0 
	warning('non-integer value entered for sv, rounding to closest integer\n');
	sv = round(sv);
end


% table of C/A Code Tap Selection (sets delay for G2 generator)
tap=[2 6;
    3 7;
    4 8;
    5 9;
    1 9;
    2 10;
    1 8;
    2 9;
    3 10;
    2 3;
    3 4;
    5 6;
    6 7;
    7 8;
    8 9;
    9 10;
    1 4;
    2 5;
    3 6;
    4 7;
    5 8;
    6 9;
    1 3;
    4 6;
    5 7;
    6 8;
    7 9;
    8 10;
    1 6;
    2 7;
    3 8;
    4 9
    5 10
    4 10
    1 7
    2 8
    4 10];

% G1 LFSR: x^10+x^3+1
s=[0 0 1 0 0 0 0 0 0 1];
n=length(s);
g1=ones(1,n);	%initialization vector for G1

%g=ones(1,38192);
%g2=ones(1,38192);
%gfs=ones(1,38192);

g=ones(1,65536/2);
g2=ones(1,65536/2);
gfs=ones(1,65536/2);

L=2^n-1;

% G2j LFSR: x^10+x^9+x^8+x^6+x^3+x^2+1
t=[0 1 1 0 0 1 0 1 1 1];
q=ones(1,n);	%initialization vector for G2

% generate C/A Code sequences:
tap_sel=tap(sv,:);
for inc=1:L
    g2(:,inc)=mod(sum(q(tap_sel),2),2);
    g(:,inc)=mod(g1(n)+g2(:,inc),2);
   g1=[mod(sum(g1.*s),2) g1(1:n-1)];
   q=[mod(sum(q.*t),2) q(1:n-1)];
end

%upsample to desired rate
if fs~=1
	%fractional upsampling with zero order hold
	index=0;
	for cnt = 1/fs:1/fs:L
		index=index+1;
		if ceil(cnt) > L   %traps a floating point error in index
			gfs(:,index)=g(:,L);
		else
			gfs(:,index)=g(:,ceil(cnt));
		end
	end 
	g=gfs;
end

== matlab function Signal_Generator/Gen 1 3/MATLAB Function ==
  data: array input; y output; shift input
function y = fcn(array, shift)

y = circshift(array, shift);

== matlab function Signal_Generator/Gen 1 2/Carrier Generator /MATLAB Function ==
  data: Frequency input; I output; time input; voltage input; Q output
function [I,Q]= fcn(Frequency, time, voltage)
u=2*pi*(Frequency+0.08*voltage)*time;
I=sin(u);
Q=cos(u);

== matlab function Signal_Generator/Gen 1 1/Carrier Generator/MATLAB Function ==
  data: Frequency input; I output; time input; voltage input; Q output
function [I,Q]= fcn(Frequency, time, voltage)
u=2*pi*(Frequency-0.04*voltage)*time;
I=sin(u);
Q=cos(u);

== matlab function Signal_Generator/Gen 1 4/Carrier Generator /MATLAB Function ==
  data: Frequency input; I output; time input; voltage input; Q output
function [I,Q]= fcn(Frequency, time, voltage)
u=2*pi*(Frequency+0.02*voltage)*time;
I=sin(u);
Q=cos(u);
